simulink model "lab7"  (R2015a)
settings: Solver=ode45  StartTime=0.0  StopTime=250.0  MaxStep=0.2  RelTol=1e-3
values from neighbouring files (symbols this model uses):
  dD = cell2mat(dD)    [lab7.m]
  ddMax = 3    [lab7.m]
  deltaMax = 30    [lab7.m]
  fConst = 0    [lab7.m]
  K = 0.08    [lab7.m]
  Kaw = 2.604    [lab7.m]
  Kc = 1.04    [lab7.m]
  nD = cell2mat(nD)    [lab7.m]
  phiZad = 90    [lab7.m]
  T = aT(i)    [lab7.m]
  Ti = 200    [lab7.m]
  Tr = 1    [lab7.m]
  Ts = 16.4    [lab7.m]
settings Model: Creator=vbox  LastModifiedBy=vbox
settings DataIOCC: InspectSignalLogs=on

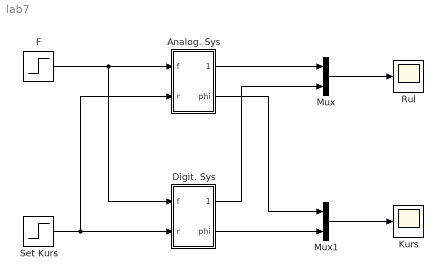
== system lab7 ==
  Analog. Sys : Subsystem
  Digit. Sys : Subsystem
  F : Step  After=fConst  SampleTime=0
  Kurs : Scope
      settings: SaveName=phi
  Mux : Mux  Inputs=2
  Mux1 : Mux  Inputs=2
  Rul : Scope
      settings: TimeRange=100  YMin=0  YMax=400  SaveName=delta
  Set Kurs : Step  Time=0  After=phiZad  SampleTime=0
  wires:
  F/1 -> Digit. Sys/1(f), Analog. Sys/1(f)
  Mux/1 -> Rul/1
  Mux1/1 -> Kurs/1
  Set Kurs/1 -> Analog. Sys/2(r), Digit. Sys/2(r)
  Analog. Sys/1(delta) -> Mux/1
  Analog. Sys/2(phi) -> Mux1/1
  Digit. Sys/2(phi) -> Mux1/2
  Digit. Sys/1(delta) -> Mux/2

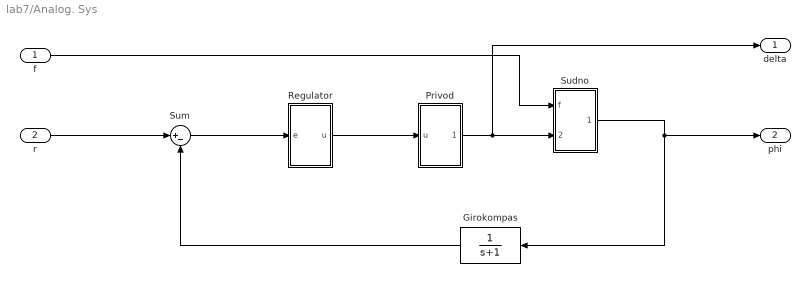
== system lab7/Analog. Sys ==
  f : Inport
  r : Inport  Port=2
  Girokompas : TransferFcn  Denominator=[1 1]
  Privod : Subsystem
  Regulator : Subsystem
  Sudno : Subsystem
  Sum : Sum  Inputs=|+-
  delta : Outport
  phi : Outport  Port=2
  wires:
  Girokompas/1 -> Sum/2
  r/1 -> Sum/1
  Sudno/1(phi) -> phi/1, Girokompas/1
  Sum/1 -> Regulator/1(e)
  f/1 -> Sudno/1(f)
  Privod/1(delta) -> delta/1, Sudno/2(delta)
  Regulator/1(u) -> Privod/1(u)

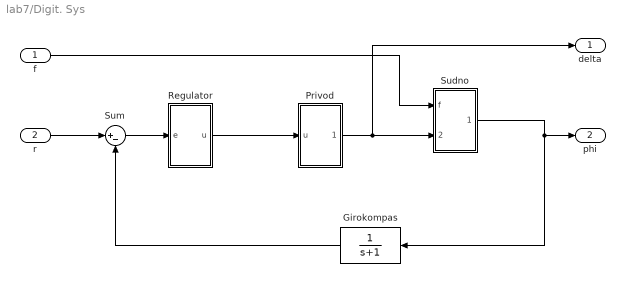
== system lab7/Digit. Sys ==
  f : Inport
  r : Inport  Port=2
  Girokompas : TransferFcn  Denominator=[1 1]
  Privod : Subsystem
  Regulator : Subsystem
  Sudno : Subsystem
  Sum : Sum  Inputs=|+-
  delta : Outport
  phi : Outport  Port=2
  wires:
  Girokompas/1 -> Sum/2
  r/1 -> Sum/1
  Sudno/1(phi) -> phi/1, Girokompas/1
  Sum/1 -> Regulator/1(e)
  f/1 -> Sudno/1(f)
  Privod/1(delta) -> delta/1, Sudno/2(delta)
  Regulator/1(u) -> Privod/1(u)

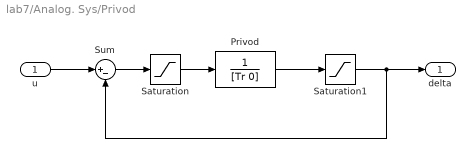
== system lab7/Analog. Sys/Privod ==
  u : Inport
  Privod : TransferFcn  Denominator=[Tr 0]
  Saturation : Saturate  UpperLimit=Tr*ddMax  LowerLimit=-Tr*ddMax
      settings: LockScale=on
  Saturation1 : Saturate  UpperLimit=deltaMax  LowerLimit=-deltaMax
  Sum : Sum  Inputs=|+-
  delta : Outport
  wires:
  u/1 -> Sum/1
  Sum/1 -> Saturation/1
  Saturation/1 -> Privod/1
  Privod/1 -> Saturation1/1
  Saturation1/1 -> Sum/2, delta/1

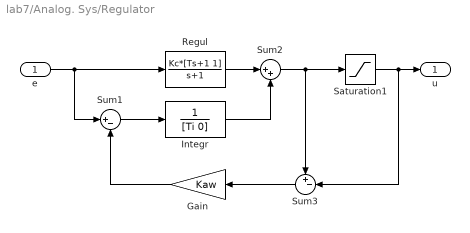
== system lab7/Analog. Sys/Regulator ==
  e : Inport
  Gain : Gain  Gain=Kaw
  Integr : TransferFcn  Denominator=[Ti 0]
  Regul : TransferFcn  Numerator=Kc*[Ts+1 1]  Denominator=[1 1]
  Saturation1 : Saturate  UpperLimit=deltaMax  LowerLimit=-deltaMax
  Sum1 : Sum  Inputs=|+-
  Sum2 : Sum  Inputs=|++
  Sum3 : Sum  Inputs=+-|
  u : Outport
  wires:
  e/1 -> Sum1/1, Regul/1
  Regul/1 -> Sum2/1
  Integr/1 -> Sum2/2
  Sum1/1 -> Integr/1
  Sum2/1 -> Saturation1/1, Sum3/1
  Saturation1/1 -> Sum3/2, u/1
  Gain/1 -> Sum1/2
  Sum3/1 -> Gain/1

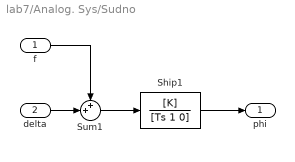
== system lab7/Analog. Sys/Sudno ==
  f : Inport
  delta : Inport  Port=2
  Ship1 : TransferFcn  Numerator=[K]  Denominator=[Ts 1 0]
  Sum1 : Sum  Inputs=++|
  phi : Outport
  wires:
  Sum1/1 -> Ship1/1
  Ship1/1 -> phi/1
  f/1 -> Sum1/1
  delta/1 -> Sum1/2

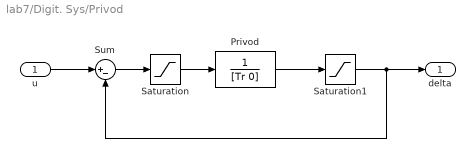
== system lab7/Digit. Sys/Privod ==
  u : Inport
  Privod : TransferFcn  Denominator=[Tr 0]
  Saturation : Saturate  UpperLimit=Tr*ddMax  LowerLimit=-Tr*ddMax
      settings: LockScale=on
  Saturation1 : Saturate  UpperLimit=deltaMax  LowerLimit=-deltaMax
  Sum : Sum  Inputs=|+-
  delta : Outport
  wires:
  u/1 -> Sum/1
  Sum/1 -> Saturation/1
  Saturation/1 -> Privod/1
  Privod/1 -> Saturation1/1
  Saturation1/1 -> Sum/2, delta/1

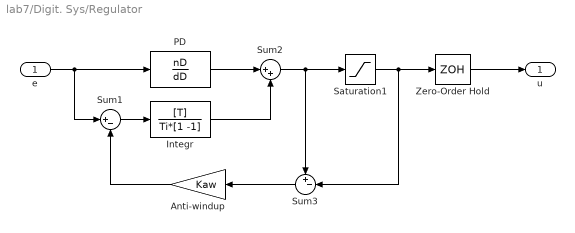
== system lab7/Digit. Sys/Regulator ==
  e : Inport
  Anti-windup : Gain  Gain=Kaw
  Integr : DiscreteTransferFcn  Numerator=[T]  Denominator=Ti*[1 -1]  SampleTime=T
  PD : DiscreteTransferFcn  Numerator=nD  Denominator=dD  SampleTime=T
  Saturation1 : Saturate  UpperLimit=deltaMax  LowerLimit=-deltaMax
  Sum1 : Sum  Inputs=|+-
  Sum2 : Sum  Inputs=|++
  Sum3 : Sum  Inputs=+-|
  Zero-Order Hold : ZeroOrderHold  SampleTime=T
  u : Outport
  wires:
  e/1 -> PD/1, Sum1/1
  Sum2/1 -> Saturation1/1, Sum3/1
  Saturation1/1 -> Zero-Order Hold/1, Sum3/2
  Anti-windup/1 -> Sum1/2
  Sum3/1 -> Anti-windup/1
  Sum1/1 -> Integr/1
  Integr/1 -> Sum2/2
  PD/1 -> Sum2/1
  Zero-Order Hold/1 -> u/1

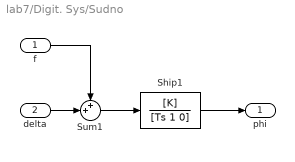
== system lab7/Digit. Sys/Sudno ==
  f : Inport
  delta : Inport  Port=2
  Ship1 : TransferFcn  Numerator=[K]  Denominator=[Ts 1 0]
  Sum1 : Sum  Inputs=++|
  phi : Outport
  wires:
  Sum1/1 -> Ship1/1
  Ship1/1 -> phi/1
  f/1 -> Sum1/1
  delta/1 -> Sum1/2
